simulink model "PVWDgridANN1"  (R2021a)
settings: Solver=VariableStepAuto  StartTime=0.0  StopTime=1  FixedStep=6.17283950617284E-7  MaxStep=2.0E-5  RelTol=1e-3
undefined symbols (not defined in the file): dEgdT, EgRef, gcbh, k1, Rsh_array5pc, sps_rtmsupport, Tref_K, VT_ref
libraries: neural x55, spsThreePhaseVIMeasurementLib x11, spsSeriesRLCBranchLib x9, spsVoltageMeasurementLib x7, spsDiodeLib x6, spsCurrentMeasurementLib x5, powerlib_extras x5, spsThreePhaseSeriesRLCBranchLib x4, spsThreePhaseBreakerLib x4, spsThreePhaseSeriesRLCLoadLib x3, spsUniversalBridgeLib x3, spsPVarrayModel x3
(part 1 of 7)
settings Model: Creator=Lenovo  LastModifiedBy=Sai Teja
settings SolverCC: AlgebraicLoopSolver=LineSearch
settings DebuggingCC: SFMachineParentedDataDiag=warning  ArithmeticOperatorsInVariantConditions=warning
settings ModelReferenceCC: EnableParallelModelReferenceBuilds=on  ModelReferenceMinAlgLoopOccurrences=on
settings SFSimCC: CustomCodeUndefinedFunction=UseInterfaceOnly

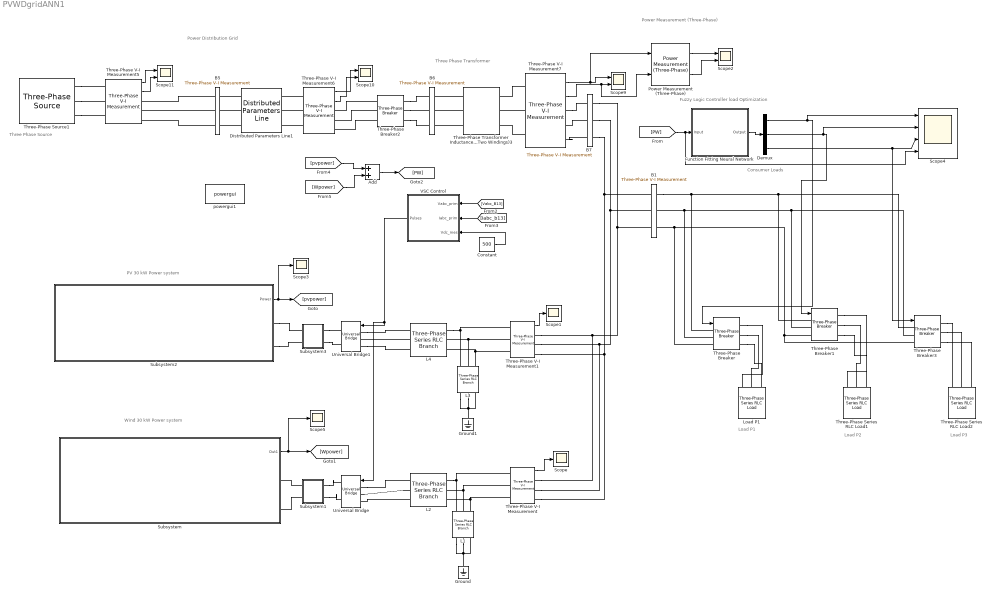
== system PVWDgridANN1 ==
  note: Fuzzy Logic Controller load Optimization
  note: Power Measurement
      | (Three-Phase)
  note: Three Phase Transformer
  note: Three Phase Source
  note: PV 30 kW Power system
  note: Load P1
  note: Power Distribution Grid
  note: Load P2
  note: Load P3
  note: Consumer Loads
  note: Wind 30 kW Power system
  Add : Sum
  B1 : spsThreePhaseVIMeasurementLib/Three-Phase V-I Measurement  VoltageMeasurement=no  SetLabelV=off  LabelV=Vabc_B13  Vpu=off  VpuLL=off  CurrentMeasurement=no  SetLabelI=off  LabelI=Iabc_b13  Ipu=off  Pbase=100e6  Vbase=440  OutputType=Magnitude  PhasorSimulation=off  PSBequivalent=0
  B5 : spsThreePhaseVIMeasurementLib/Three-Phase V-I Measurement  VoltageMeasurement=no  SetLabelV=off  LabelV=Vabc_B12  Vpu=off  VpuLL=off  CurrentMeasurement=no  SetLabelI=off  LabelI=A1  Ipu=off  Pbase=100e6  Vbase=25e3  OutputType=Magnitude  PhasorSimulation=off  PSBequivalent=0
  B6 : spsThreePhaseVIMeasurementLib/Three-Phase V-I Measurement  VoltageMeasurement=no  SetLabelV=off  LabelV=Vabc_B12  Vpu=off  VpuLL=off  CurrentMeasurement=no  SetLabelI=off  LabelI=A1  Ipu=off  Pbase=100e6  Vbase=440  OutputType=Magnitude  PhasorSimulation=off  PSBequivalent=0
  B7 : spsThreePhaseVIMeasurementLib/Three-Phase V-I Measurement  VoltageMeasurement=phase-to-ground  SetLabelV=on  LabelV=Vabc_B13  Vpu=off  VpuLL=off  CurrentMeasurement=yes  SetLabelI=on  LabelI=Iabc_b13  Ipu=off  Pbase=100e6  Vbase=440  OutputType=Magnitude  PhasorSimulation=off  PSBequivalent=0
  Constant : Constant  Value=500
  Demux : Demux  Outputs=3
  Distributed Parameters Line1 : spsDistributedParametersLineLib/Distributed Parameters Line  Phases=3  Length=100  Frequency=50  Resistance=[0.01273 0.3864]  Inductance="[0.9337e-3  4.1264e-3]"  Capacitance=[12.74e-9 7.751e-9]  x1=[-0.0006 1.14367698661715e-09 21086.3723397964 -61017.1446248442;-0.0005 1.07493118065828e-09 22992.5623173876 -60324.6973859194;-0.0004 1.00512454740211e-09 24876.0614118971 -59572.7169537636;-0.0003 9.34325977567818e-10 26735.0108371164 -58761.9454422758;-0.0002 8.62605340796205e-10 28567.5760343965 -57893.1829850521;-0.0001 7.90033416696831e-10 30371.9484831358 -56967.2869457508]  x2=[-0.0006 5.86941597339754e-09 21194.91938393 -61383.6988829109;-0.0005 5.59404825033619e-09 23112.5695475968 -60687.6612265351;-0.0004 5.31315987702939e-09 25007.4103955344 -59931.7321754389;-0.0003 5.02702805638952e-09 26877.5719485928 -59116.6577403313;-0.0002 4.73593516597845e-09 28721.2085831066 -58243.2423012745;-0.0001 4.44016847933494e-09 30536.5008523023 -57312.3478138583]  x3=[-0.0006 5.6514601122434e-11 53.1137000849838 -233.04087477199;-0.0005 5.70127645300196e-11 60.4074824530608 -231.25754153085;-0.0004 5.74546632222485e-11 67.6416499290405 -229.245985016281;-0.0003 5.78398610984626e-11 74.8090632630155 -227.008190391703;-0.0002 5.81679780148637e-11 81.9026490833576 -224.54636609024;-0.0001 5.84386901596691e-11 88.9154068772811 -221.862941635257]  x4=[-0.0006 -4.63263341454855e-11 78.0562173688537 -225.948056909574;-0.0005 -4.72451010975785e-11 85.1149013172606 -223.384760144692;-0.0004 -4.81172428388583e-11 92.089587134114 -220.601009591115;-0.0003 -4.89418986707213e-11 98.9733916465766 -217.599552474555;-0.0002 -4.97182547574234e-11 105.759521370686 -214.383350870815;-0.0001 -5.04455449292375e-11 112.441279215705 -210.955578782581]  x5=0.000565541566995743  V1=[0 0 0 1.442e-09 6.456e+04 6.456e+04;0 0 0 314.2 314.2 314.2;1.571 1.571 1.571 -0.8406 0.4129 -1.158]  V2=[0 0 0 6.152e-09 6.494e+04 6.494e+04;0 0 0 314.2 314.2 314.2;1.571 1.571 1.571 -0.9733 0.4126 -1.158]  I1=[0 0 0 3.485e-11 239 239;0 0 0 314.2 314.2 314.2;1.571 1.571 1.571 -2.244 0.3044 -1.266]  I2=[0 0 0 3.246e-11 239 239;0 0 0 314.2 314.2 314.2;1.571 1.571 1.571 0.613 0.4126 -1.158]  nHarmo=2  Measurements=None  Decoupling=off  VsMag0=0  VrMag0=0  VsAngle0=0  VrAngle0=0  IsMag0=0  IrMag0=0  IsAngle0=0  IrAngle0=0
      settings: SourceProductBaseCode=PS
  Function Fitting Neural Network : Subsystem
      mask help: Function Fitting Neural Network
      mask Display: e = 0.06;c1 = [120 150 230]/255;c2 = ([120 150 230]+0)/383;c3 = ([120 150 230]+128)/383;patch([0 1 1 0],[0 0 1 1],c1);patch([0 1 1 1-e 1-e 0+e],[0 0 1 1-e 0+e 0+e],c2);patch([0 0 1 1-e 0+e 0+e],[0 1 1 1-e 1-e 0+e],c3);plot([0 1 1 0 0],[0 0 1 1 0]);fprintf('NNET');port_label('input',1,' Input');port_label('output',1,'Output ');
  Ground : spsGroundLib/Ground  LConnTagsString=a
  Ground1 : spsGroundLib/Ground  LConnTagsString=a
  L1 : spsThreePhaseSeriesRLCBranchLib/Three-Phase Series RLC Branch  LConnTagsString=A|B|C  RConnTagsString=A|B|C  BranchType=C  Resistance=500e-6*377/50/2  Inductance=1e-2  Capacitance=100e-6  Measurements=None
  L2 : spsThreePhaseSeriesRLCBranchLib/Three-Phase Series RLC Branch  LConnTagsString=A|B|C  RConnTagsString=A|B|C  BranchType=RL  Resistance=1  Inductance=3e-2  Capacitance=900e-6  Measurements=None
  L3 : spsThreePhaseSeriesRLCBranchLib/Three-Phase Series RLC Branch  LConnTagsString=A|B|C  RConnTagsString=A|B|C  BranchType=C  Resistance=500e-6*377/50/2  Inductance=1e-2  Capacitance=100e-6  Measurements=None
  L4 : spsThreePhaseSeriesRLCBranchLib/Three-Phase Series RLC Branch  LConnTagsString=A|B|C  RConnTagsString=A|B|C  BranchType=RL  Resistance=1  Inductance=3e-2  Capacitance=900e-6  Measurements=None
  Load P1 : spsThreePhaseSeriesRLCLoadLib/Three-Phase Series RLC Load  LConnTagsString=A|B|C  Configuration=Y (grounded)  NominalVoltage=400  Vabc=[1e3 1e3 1e3]  Vabcp=[1e3 1e3 1e3]  NominalFrequency=50  UnbalancedPower=off  ActivePower=10e3  InductivePower=100  CapacitivePower=0  Pabc=[10e3 9e3 11e3]  QLabc=[100 90 110]  QCabc=[100 90 110]  Pabcp=[10e3 9e3 11e3]  QLabcp=[100 90 110]  QCabcp=[100 90 110]  Measurements=None  LoadType=constant Z
  Power Measurement (Three-Phase) : eePowerMeasurement/Power Measurement (Three-Phase)  LabelModeActiveChoice=Continuous  F=60  K=[0 1 2 3]  Seq=Positive  Ts=0
      settings: SourceProductBaseCode=PS
  Scope{,1,3,5} (4 alike) : Scope
  Scope{2,9..11} (4 alike) : Scope  NumInputPorts=2
  Scope4 : Scope  NumInputPorts=4
  Subsystem : Subsystem
  Subsystem1 : Subsystem
  Subsystem2 : Subsystem
  Subsystem3 : Subsystem
  Three-Phase Series RLC Load1 : spsThreePhaseSeriesRLCLoadLib/Three-Phase Series RLC Load  LConnTagsString=A|B|C  Configuration=Y (grounded)  NominalVoltage=400  Vabc=[1e3 1e3 1e3]  Vabcp=[1e3 1e3 1e3]  NominalFrequency=50  UnbalancedPower=off  ActivePower=10e3  InductivePower=100  CapacitivePower=0  Pabc=[10e3 9e3 11e3]  QLabc=[100 90 110]  QCabc=[100 90 110]  Pabcp=[10e3 9e3 11e3]  QLabcp=[100 90 110]  QCabcp=[100 90 110]  Measurements=None  LoadType=constant Z
  Three-Phase Series RLC Load2 : spsThreePhaseSeriesRLCLoadLib/Three-Phase Series RLC Load  LConnTagsString=A|B|C  Configuration=Y (grounded)  NominalVoltage=400  Vabc=[1e3 1e3 1e3]  Vabcp=[1e3 1e3 1e3]  NominalFrequency=50  UnbalancedPower=off  ActivePower=10e3  InductivePower=100  CapacitivePower=0  Pabc=[10e3 9e3 11e3]  QLabc=[100 90 110]  QCabc=[100 90 110]  Pabcp=[10e3 9e3 11e3]  QLabcp=[100 90 110]  QCabcp=[100 90 110]  Measurements=None  LoadType=constant Z
  Three-Phase V-I Measurement : spsThreePhaseVIMeasurementLib/Three-Phase V-I Measurement  VoltageMeasurement=phase-to-phase  SetLabelV=off  LabelV=Vabc  Vpu=off  VpuLL=off  CurrentMeasurement=no  SetLabelI=off  LabelI=Iabc  Ipu=off  Pbase=100e6  Vbase=500e3  OutputType=Complex  PhasorSimulation=off  PSBequivalent=0
  Three-Phase V-I Measurement1 : spsThreePhaseVIMeasurementLib/Three-Phase V-I Measurement  VoltageMeasurement=phase-to-phase  SetLabelV=off  LabelV=Vabc  Vpu=off  VpuLL=off  CurrentMeasurement=no  SetLabelI=off  LabelI=Iabc  Ipu=off  Pbase=100e6  Vbase=500e3  OutputType=Complex  PhasorSimulation=off  PSBequivalent=0
  Three-Phase V-I Measurement5 : spsThreePhaseVIMeasurementLib/Three-Phase V-I Measurement  VoltageMeasurement=phase-to-ground  SetLabelV=off  LabelV=Vabc  Vpu=off  VpuLL=off  CurrentMeasurement=yes  SetLabelI=off  LabelI=Iabc  Ipu=off  Pbase=100e6  Vbase=500e3  OutputType=Complex  PhasorSimulation=off  PSBequivalent=0
  Three-Phase V-I Measurement6 : spsThreePhaseVIMeasurementLib/Three-Phase V-I Measurement  VoltageMeasurement=phase-to-ground  SetLabelV=off  LabelV=Vabc  Vpu=off  VpuLL=off  CurrentMeasurement=yes  SetLabelI=off  LabelI=Iabc  Ipu=off  Pbase=100e6  Vbase=500e3  OutputType=Complex  PhasorSimulation=off  PSBequivalent=0
  Three-Phase V-I Measurement7 : spsThreePhaseVIMeasurementLib/Three-Phase V-I Measurement  VoltageMeasurement=phase-to-phase  SetLabelV=off  LabelV=Vabc_b1  Vpu=off  VpuLL=off  CurrentMeasurement=yes  SetLabelI=off  LabelI=Iabc_b1  Ipu=off  Pbase=100e6  Vbase=500e3  OutputType=Complex  PhasorSimulation=off  PSBequivalent=0
  Three-Phase Breaker : spsThreePhaseBreakerLib/Three-Phase Breaker  InitialState=open  SwitchA=on  SwitchB=on  SwitchC=on  SwitchTimes="[1/60  5/60]"  External=on  BreakerResistance=0.01  SnubberResistance=1e6  SnubberCapacitance=inf  Measurements=None
  Three-Phase Breaker1 : spsThreePhaseBreakerLib/Three-Phase Breaker  InitialState=open  SwitchA=on  SwitchB=on  SwitchC=on  SwitchTimes="[1/60  5/60]"  External=on  BreakerResistance=0.01  SnubberResistance=1e6  SnubberCapacitance=inf  Measurements=None
  Three-Phase Breaker2 : spsThreePhaseBreakerLib/Three-Phase Breaker  InitialState=closed  SwitchA=off  SwitchB=off  SwitchC=off  SwitchTimes="[1/50  20/50]"  External=off  BreakerResistance=0.001  SnubberResistance=1e6  SnubberCapacitance=inf  Measurements=None
  Three-Phase Breaker3 : spsThreePhaseBreakerLib/Three-Phase Breaker  InitialState=open  SwitchA=on  SwitchB=on  SwitchC=on  SwitchTimes="[1/60  5/60]"  External=on  BreakerResistance=0.01  SnubberResistance=1e6  SnubberCapacitance=inf  Measurements=None
  Three-Phase Source1 : spsThreePhaseSourceLib/Three-Phase Source  InternalConnection=Yg  VoltagePhases=off  Voltage=63510.4  PhaseAngle=0  Voltage_phases=[25e3 25e3 25e3]/sqrt(3)  PhaseAngles_phases=[0 -120 +120]  Frequency=50  NonIdealSource=on  SpecifyImpedance=on  Resistance=0.8929  Inductance=16.58e-3  ShortCircuitLevel=100e6  BaseVoltage=63510.4  XRratio=7  BusType=swing  Pref=0  Qref=0  Prefabc=[10e3, 10e3, 10e3]  Qrefabc=[0, 0, 0]  Qmin=-inf  Qmax=inf
  Three-Phase Transformer Inductance Matrix Type (Two Windings)3 : spsThreePhaseTransformerInductanceMatrixTypeTwoWindingsLib/Three-Phase Transformer Inductance Matrix Type (Two Windings)  CoreType=Three-limb or five-limb core  Winding1Connection=Yg  Winding2Connection=Yg  AutoTransformer=off  Measurements=None  NominalPower=[100e3 50]  VLLnom=[63510.4 254.03]  WindingResistances=[0.01 0.01]  NoLoadIexcPos=2  NoLoadPlossPos=1000  ShortCircuitReactancePos=0.06  ShortCircuitReactancePosAuto=0.06  NoLoadIexcZero=100  NoLoadPlossZero=1500  ShortCircuitReactanceZero=0.03  ShortCircuitReactanceZeroAuto=0.03
      settings: SourceProductBaseCode=PS
  Universal Bridge : spsUniversalBridgeLib/Universal Bridge  Arms=3  SnubberResistance=1e5  SnubberCapacitance=inf  Device=MOSFET / Diodes  Ron=1e-3  Lon=0  ForwardVoltages="[  0  0  ]"  ForwardVoltage=0  GTOparameters=[ 10e-6 , 20e-6 ]  IGBTparameters=[ 1e-6 , 2e-6 ]  Measurements=None  Measurements_2=None  converterType=Rectifier
  Universal Bridge1 : spsUniversalBridgeLib/Universal Bridge  Arms=3  SnubberResistance=1e5  SnubberCapacitance=inf  Device=MOSFET / Diodes  Ron=1e-3  Lon=0  ForwardVoltages="[  0  0  ]"  ForwardVoltage=0  GTOparameters=[ 10e-6 , 20e-6 ]  IGBTparameters=[ 1e-6 , 2e-6 ]  Measurements=None  Measurements_2=None  converterType=Rectifier
  VSC Control : Subsystem  mask(VSC Main Controller){nom=[ 100e3  50 ], Vnom=[ 440 440 ], Vnom_dc=440, RLxfo=[0.002  0.06 ], RLchoke=[2e-3  250e-6  ], K_VDCreg=[7  800], K_Ireg=[0.3 20], Ts=50e-6}
      mask prompts: nom "Nominal power and frequency [ Pnom(VA)  Fnom(Hz) ]:"; Vnom "Nominal primary and secondary voltages (Vrms LL) [ Vnom_prim   Vnom_sec ]:"; Vnom_dc "Nominal DC bus voltage (V):"; RLxfo "Total transformer leakage impedance (pu/Pnom) [ Rxfo  Lxf ]"; RLchoke "Choke impedance [ R(ohm) L(H) ]"; K_VDCreg "VDC regultator gains [ Kp  Ki ]:"; K_Ireg "Current regulator gains [ Kp  Ki ]:"; Ts "Sample time"
      mask init:
      | Pnom=nom(1);
      | Fnom=nom(2);
      | Vnom_prim=Vnom(1);
      | Vnom_sec=Vnom(2);
      | Zbase=Vnom_sec^2/Pnom;
      | Rtot_pu=RLxfo(1) + RLchoke(1)/Zbase;
      | Ltot_pu=RLxfo(2) + RLchoke(2)/(Zbase/(2*pi*Fnom));
      | Kp_VDCreg=K_VDCreg(1);
      | Ki_VDCreg=K_VDCreg(2);
      | Kp_Ireg=K_Ireg(1);
      | Ki_Ireg=K_Ireg(2);
      | Vdc_ref=Vnom_dc;
      | % Used to determine initial value of Boost Control (MPPT)
      | assignin('base','Vdc_ref_Inv',Vdc_ref);
  powergui1 : spspowerguiLib/powergui  Priority=1  SimulationMode=Discrete  SampleTime=1e-4  frequency=60  Iterations=50  frequencyindice=50  Pbase=100e6  ErrMax=1e-4  UnitsV=kV  UnitsW=MW  buscounter=0  FunctionMessages=off  echomessages=off  EnableUseOfTLC=off  CurrentSourceSwitches=off  DisableSnubberDevices=off  DisableRonSwitches=off  DisableVfSwitches=off  DisplayEquations=off  AutomaticDiscreteSolvers=off  SolverType=Tustin/Backward Euler (TBE)  Interpol=off  ExternalGateDelay=off  methode=off  Ts=100  x0status=blocks  SPID=on  SwTol=0  HookPort=off  NonlinearTolerance=0  nMaxIteration=15  ContinueOnMaxIteration=off  RestoreLinks=warning  ResistiveCurrentMeasurement=off  Frange=[0:2:500]  Ylog=off  Xlog=on  ShowGrid=off  save=off  variable=ZData  structure=Ctrl_Sig  ZoomFFT=off  StartTime=0.0  cycles=1  DisplayStyle=1  fundamental=60  FreqAxis=off  MaxFrequency=1000  frequencyindicesteady=1  RmsSteady=1  display=off
  wires:
  Three-Phase V-I Measurement5/2 -> Scope11/2
  Three-Phase V-I Measurement5/1 -> Scope11/1
  Three-Phase V-I Measurement7/1 -> Power Measurement (Three-Phase)/1, Scope9/1
  Three-Phase V-I Measurement6/2 -> Scope10/2
  Three-Phase V-I Measurement6/1 -> Scope10/1
  [Vabc_B13] -> VSC Control/1(Vabc_prim)
  [Iabc_b13] -> VSC Control/2(Iabc_prim)
  Constant/1 -> VSC Control/3(Vdc_mes)
  VSC Control/1(Pulses) -> Universal Bridge/1, Universal Bridge1/1
  Three-Phase V-I Measurement1/1 -> Scope1/1
  Three-Phase V-I Measurement7/2 -> Power Measurement (Three-Phase)/2, Scope9/2
  Power Measurement (Three-Phase)/1 -> Scope2/1
  Power Measurement (Three-Phase)/2 -> Scope2/2
  Function Fitting Neural Network/1(Output) -> Demux/1
  Demux/1 -> Scope4/1, Three-Phase Breaker/1
  Demux/2 -> Scope4/2, Three-Phase Breaker1/1
  Subsystem2/1(Power) -> Scope3/1, [pvpower]
  [PW] -> Scope4/4, Function Fitting Neural Network/1(Input)
  Demux/3 -> Three-Phase Breaker3/1, Scope4/3
  Subsystem/1(Out1) -> [Wpower], Scope5/1
  Three-Phase V-I Measurement/1 -> Scope/1
  [pvpower] -> Add/1
  [Wpower] -> Add/2
  Add/1 -> [PW]
  connections:
  B5/RConn2 -- Three-Phase V-I Measurement5/RConn2
  Three-Phase Breaker2/LConn2 -- B6/RConn2
  Three-Phase Source1/RConn2 -- Three-Phase V-I Measurement5/LConn2
  Three-Phase V-I Measurement7/RConn3 -- B7/RConn3
  B5/RConn1 -- Three-Phase V-I Measurement5/RConn1
  Three-Phase V-I Measurement6/LConn1 -- Distributed Parameters Line1/RConn1
  Three-Phase Breaker2/RConn3 -- Three-Phase V-I Measurement6/RConn3
  Three-Phase V-I Measurement7/LConn3 -- Three-Phase Transformer Inductance Matrix Type (Two Windings)3/RConn3
  Three-Phase V-I Measurement7/LConn2 -- Three-Phase Transformer Inductance Matrix Type (Two Windings)3/RConn2
  Three-Phase Transformer Inductance Matrix Type (Two Windings)3/LConn2 -- B6/LConn2
  Three-Phase Breaker2/LConn1 -- B6/RConn1
  Three-Phase Source1/RConn3 -- Three-Phase V-I Measurement5/LConn3
  Three-Phase V-I Measurement7/RConn2 -- B7/RConn2
  B5/RConn3 -- Three-Phase V-I Measurement5/RConn3
  Three-Phase V-I Measurement6/LConn3 -- Distributed Parameters Line1/RConn3
  Distributed Parameters Line1/LConn2 -- B5/LConn2
  Three-Phase Breaker2/RConn2 -- Three-Phase V-I Measurement6/RConn2
  Distributed Parameters Line1/LConn3 -- B5/LConn3
  Three-Phase V-I Measurement6/LConn2 -- Distributed Parameters Line1/RConn2
  Distributed Parameters Line1/LConn1 -- B5/LConn1
  Three-Phase Source1/RConn1 -- Three-Phase V-I Measurement5/LConn1
  Three-Phase V-I Measurement7/RConn1 -- B7/RConn1
  Three-Phase Breaker2/RConn1 -- Three-Phase V-I Measurement6/RConn1
  Three-Phase Transformer Inductance Matrix Type (Two Windings)3/LConn1 -- B6/LConn1
  Three-Phase Breaker2/LConn3 -- B6/RConn3
  Three-Phase Transformer Inductance Matrix Type (Two Windings)3/LConn3 -- B6/LConn3
  Three-Phase V-I Measurement7/LConn1 -- Three-Phase Transformer Inductance Matrix Type (Two Windings)3/RConn1
  B7/LConn3 -- Three-Phase V-I Measurement/RConn3 -- Three-Phase V-I Measurement1/RConn3 -- B1/RConn1
  B7/LConn2 -- Three-Phase V-I Measurement/RConn2 -- Three-Phase V-I Measurement1/RConn2 -- B1/RConn2
  B7/LConn1 -- Three-Phase V-I Measurement/RConn1 -- Three-Phase V-I Measurement1/RConn1 -- B1/RConn3
  L3/LConn3 -- Three-Phase V-I Measurement1/LConn3 -- L4/RConn3
  L3/LConn1 -- L4/RConn1 -- Three-Phase V-I Measurement1/LConn1
  L3/LConn2 -- Three-Phase V-I Measurement1/LConn2 -- L4/RConn2
  L3/RConn1 -- Ground1/LConn1 -- L3/RConn3 -- L3/RConn2
  L4/LConn2 -- Universal Bridge1/LConn2
  Universal Bridge1/LConn3 -- L4/LConn3
  Subsystem3/RConn1 -- Universal Bridge1/RConn1
  Subsystem3/RConn2 -- Universal Bridge1/RConn2
  Universal Bridge1/LConn1 -- L4/LConn1
  Subsystem2/RConn1 -- Subsystem3/LConn1
  Subsystem2/RConn2 -- Subsystem3/LConn2
  Three-Phase Breaker/RConn1 -- Load P1/LConn1
  Three-Phase Breaker/RConn2 -- Load P1/LConn2
  Three-Phase Breaker/RConn3 -- Load P1/LConn3
  Three-Phase Breaker1/RConn3 -- Three-Phase Series RLC Load1/LConn3
  Three-Phase Breaker1/RConn1 -- Three-Phase Series RLC Load1/LConn1
  Three-Phase Breaker1/RConn2 -- Three-Phase Series RLC Load1/LConn2
  Three-Phase Breaker3/RConn1 -- Three-Phase Series RLC Load2/LConn1
  Three-Phase Breaker3/RConn3 -- Three-Phase Series RLC Load2/LConn3
  Three-Phase Breaker3/RConn2 -- Three-Phase Series RLC Load2/LConn2
  B1/LConn1 -- Three-Phase Breaker/LConn1 -- Three-Phase Breaker1/LConn1 -- Three-Phase Breaker3/LConn1
  Three-Phase Breaker3/LConn2 -- Three-Phase Breaker1/LConn2 -- Three-Phase Breaker/LConn2 -- B1/LConn2
  Three-Phase Breaker3/LConn3 -- Three-Phase Breaker/LConn3 -- B1/LConn3 -- Three-Phase Breaker1/LConn3
  L2/RConn2 -- L1/LConn2 -- Three-Phase V-I Measurement/LConn2
  L2/RConn3 -- L1/LConn3 -- Three-Phase V-I Measurement/LConn3
  L1/LConn1 -- L2/RConn1 -- Three-Phase V-I Measurement/LConn1
  L1/RConn3 -- L1/RConn1 -- Ground/LConn1 -- L1/RConn2
  Subsystem1/LConn2 -- Subsystem/RConn2
  Subsystem1/RConn1 -- Universal Bridge/RConn1
  Subsystem1/LConn1 -- Subsystem/RConn1
  Universal Bridge/LConn1 -- L2/LConn1
  Subsystem1/RConn2 -- Universal Bridge/RConn2
  L2/LConn2 -- Universal Bridge/LConn2
  Universal Bridge/LConn3 -- L2/LConn3

== system PVWDgridANN1/Function Fitting Neural Network ==
  Input : Inport  PortDimensions=1
      mask Display: e = 0.06;c1 = [120 230 180]/255;c2 = ([120 230 180]+0)/(256+128);c3 = ([120 230 180]+128)/(256+128);patch([0 1 1 0],[0 0 1 1],c1);patch([0 1 1 1-e 1-e 0+e],[0 0 1 1-e 0+e 0+e],c2);patch([0 0 1 1-e 0+e 0+e],[0 1 1 1-e 1-e 0+e],c3);plot([0 1 1 0 0],[0 0 1 1 0]);
  Layer 1 : Subsystem
      mask Display: e = 0.06;c1 = [120 150 230]/255;c2 = ([120 150 230]+0)/383;c3 = ([120 150 230]+128)/383;patch([0 1 1 0],[0 0 1 1],c1);patch([0 1 1 1-e 1-e 0+e],[0 0 1 1-e 0+e 0+e],c2);patch([0 0 1 1-e 0+e 0+e],[0 1 1 1-e 1-e 0+e],c3);plot([0 1 1 0 0],[0 0 1 1 0]);
  Layer 2 : Subsystem
      mask Display: e = 0.06;c1 = [120 150 230]/255;c2 = ([120 150 230]+0)/383;c3 = ([120 150 230]+128)/383;patch([0 1 1 0],[0 0 1 1],c1);patch([0 1 1 1-e 1-e 0+e],[0 0 1 1-e 0+e 0+e],c2);patch([0 0 1 1-e 0+e 0+e],[0 1 1 1-e 1-e 0+e],c3);plot([0 1 1 0 0],[0 0 1 1 0]);
  Process Input 1 : Subsystem
      mask Display: e = 0.06;c1 = [120 150 230]/255;c2 = ([120 150 230]+0)/383;c3 = ([120 150 230]+128)/383;patch([0 1 1 0],[0 0 1 1],c1);patch([0 1 1 1-e 1-e 0+e],[0 0 1 1-e 0+e 0+e],c2);patch([0 0 1 1-e 0+e 0+e],[0 1 1 1-e 1-e 0+e],c3);plot([0 1 1 0 0],[0 0 1 1 0]);
  Output : Outport  InitialOutput=[0;0;0]
      mask Display: e = 0.06;c1 = [120 230 180]/255;c2 = ([120 230 180]+0)/(256+128);c3 = ([120 230 180]+128)/(256+128);patch([0 1 1 0],[0 0 1 1],c1);patch([0 1 1 1-e 1-e 0+e],[0 0 1 1-e 0+e 0+e],c2);patch([0 0 1 1-e 0+e 0+e],[0 1 1 1-e 1-e 0+e],c3);plot([0 1 1 0 0],[0 0 1 1 0]);
  wires:
  Input/1 -> Process Input 1/1(x)
  Layer 2/1("a{2}") -> Output/1
  Process Input 1/1(p) -> Layer 1/1("p{1}")
  Layer 1/1("a{1}") -> [feedback1]
  [feedback1] -> Layer 2/1("a{1} ")

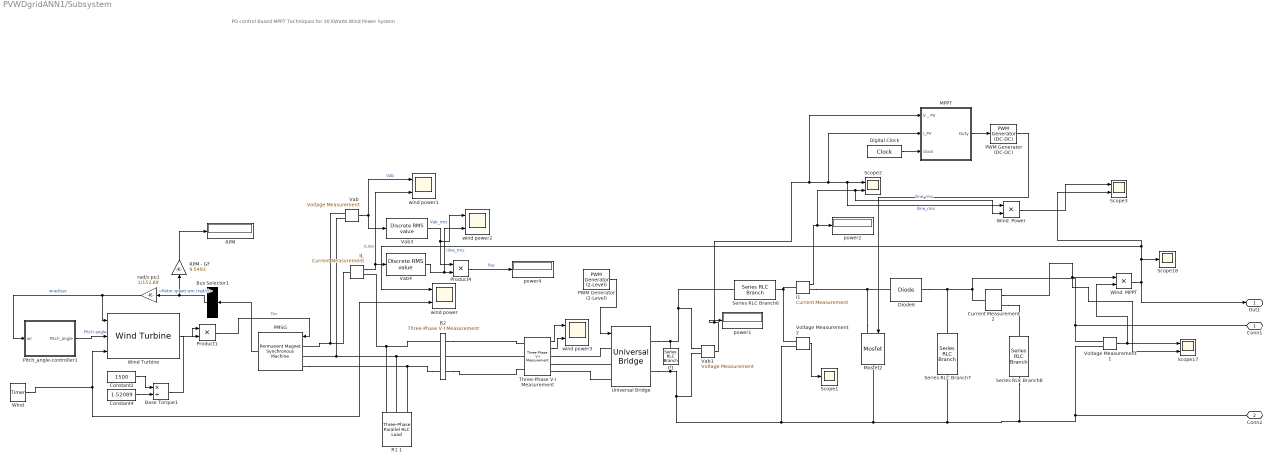
== system PVWDgridANN1/Subsystem ==
  note: PO control Based MPPT Techniques for 30 KWatts Wind Power System
  "B2 " : spsThreePhaseVIMeasurementLib/Three-Phase V-I Measurement  VoltageMeasurement=no  SetLabelV=on  LabelV=Vabc_B2  Vpu=off  VpuLL=off  CurrentMeasurement=no  SetLabelI=on  LabelI=Iabc_B2  Ipu=off  Pbase=100e6  Vbase=500e3  OutputType=Magnitude  PhasorSimulation=off  PSBequivalent=0
  Base Torque1 : Product  Inputs=*/  RndMeth=Zero
  Bus Selector1 : BusSelector  OutputSignals=Rotor speed wm (rad/s)
  C1 : spsSeriesRLCBranchLib/Series RLC Branch  LConnTagsString=__new0  RConnTagsString=__new0  BranchType=C  Resistance=0.001  Inductance=1e-3  SetiL0=off  InitialCurrent=0  Capacitance=900e-6  Setx0=off  InitialVoltage=0  Measurements=None
  Constant2 : Constant  Value=1500
  Constant4 : Constant  Value=1.52089
  Current Measurement2 : spsCurrentMeasurementLib/Current Measurement  PhasorSimulation=off  OutputType=Complex  PSBequivalent=0
  Digital Clock : DigitalClock  SampleTime=0.001
  Diode6 : spsDiodeLib/Diode  Ron=0.001  Lon=0  Vf=0.8  IC=0  UseSnubber=0  Rs=500  Cs=250e-9  Measurements=off
  I1 : spsCurrentMeasurementLib/Current Measurement  PhasorSimulation=off  OutputType=Complex  PSBequivalent=0
  IL : spsCurrentMeasurementLib/Current Measurement  PhasorSimulation=off  OutputType=Complex  PSBequivalent=0
  MPPT : Subsystem
  Mosfet2 : spsMosfetLib/Mosfet  Ron=0.1  Lon=0  Rd=0.01  Vfd=0.8  IC=0  Rs=1e5  Cs=inf  Measurements=off
  PMSG : spsPermanentMagnetSynchronousMachineLib/Permanent Magnet Synchronous Machine  NbPhases=3  FluxDistribution=Sinusoidal  RotorType=Round  MechanicalLoad=Torque Tm  PresetModel="16:  111 Nm 560 Vdc 3000 RPM - 126 Nm"  ShowDetailedParameters=on  MeasurementBus=off  Resistance=0.05  Inductance=8.5e-3  dqInductances=[0.0082 0.0082]  La=0.000635  MachineConstant=Flux linkage established by magnets (V.s)  Flux=0.192  VoltageCst=139.2998  TorqueCst=1.152  Flat=120  Mechanical=[0.011 0.001889 4 0]  PolePairs=4  InitialConditions=[0,0, 0,0]  InitialConditions5ph=[0 0 0 0 0 0]  RefAngle=90 degrees behind phase A axis (modified Park)  IterativeDiscreteModel=Trapezoidal non iterative  TsBlock=-1  TsPowergui=0
  PWM Generator (2-Level) : spsPWMGenerator2LevelLib/PWM Generator (2-Level)  ModulatorType=Three-phase bridge (6 pulses)  ModulatorMode=Unsynchronized  Fc=3000  Pc=90  nF=27  MinMax="[ -1  1 ]"  SamplingTechnique=Natural  ModulatingSignals=on  m=0.8  Freq=50  Phase=0  Ts=0  ShowCarrierOutport=off
  PWM Generator (DC-DC) : spsPWMGeneratorDCDCLib/PWM Generator (DC-DC)  Fsw=5000  Ts=0
  Pitch_angle-controller1 : Subsystem
  Product1 : Product  RndMeth=Zero
  Product4 : Product  RndMeth=Zero
  R1 1 : spsThreePhaseParallelRLCLoadLib/Three-Phase Parallel RLC Load  LConnTagsString=A|B|C  Configuration=Y (grounded)  NominalVoltage=220  Vabc=[1e3 1e3 1e3]  Vabcp=[1e3 1e3 1e3]  NominalFrequency=50  UnbalancedPower=off  ActivePower=5000  InductivePower=0  CapacitivePower=0  Pabc=[9e3 9e3 9e3]  QLabc=[100 90 110]  QCabc=[100 90 110]  Pabcp=[10e3 9e3 11e3]  QLabcp=[100 90 110]  QCabcp=[100 90 110]  Measurements=None  LoadType=constant Z
  "RPM " : Display
  RPM - GF : Gain  Gain=9.5493  SaturateOnIntegerOverflow=on  OutDataTypeStr=Inherit: Same as input  ParamDataTypeStr=Inherit: Same as input
  Scope1 : Scope
  Scope17 : Scope  NumInputPorts=2
  Scope18 : Scope
  Scope2 : Scope  NumInputPorts=2
  Scope3 : Scope  NumInputPorts=2
  Series RLC Branch6 : spsSeriesRLCBranchLib/Series RLC Branch  LConnTagsString=__new0  RConnTagsString=__new0  BranchType=L  Resistance=1  Inductance=0.4e-1  SetiL0=off  InitialCurrent=0  Capacitance=1e-6  Setx0=off  InitialVoltage=0  Measurements=None
  Series RLC Branch7 : spsSeriesRLCBranchLib/Series RLC Branch  LConnTagsString=__new0  RConnTagsString=__new0  BranchType=C  Resistance=110  Inductance=1e-3  SetiL0=off  InitialCurrent=0  Capacitance=750e-6  Setx0=off  InitialVoltage=0  Measurements=None
  Series RLC Branch8 : spsSeriesRLCBranchLib/Series RLC Branch  LConnTagsString=__new0  RConnTagsString=__new0  BranchType=R  Resistance=6  Inductance=1e-3  SetiL0=off  InitialCurrent=0  Capacitance=1e-6  Setx0=off  InitialVoltage=0  Measurements=None
  Three-Phase V-I Measurement : spsThreePhaseVIMeasurementLib/Three-Phase V-I Measurement  VoltageMeasurement=phase-to-phase  SetLabelV=off  LabelV=Vabc  Vpu=off  VpuLL=off  CurrentMeasurement=yes  SetLabelI=off  LabelI=Iabc  Ipu=off  Pbase=100e6  Vbase=500e3  OutputType=Complex  PhasorSimulation=off  PSBequivalent=0
  Universal Bridge : spsUniversalBridgeLib/Universal Bridge  Arms=3  SnubberResistance=1e5  SnubberCapacitance=inf  Device=Thyristors  Ron=1e-3  Lon=0  ForwardVoltages="[  0  0  ]"  ForwardVoltage=0.8  GTOparameters=[ 10e-6 , 20e-6 ]  IGBTparameters=[ 1e-6 , 2e-6 ]  Measurements=None  Measurements_2=None  converterType=Rectifier
  Vab : spsVoltageMeasurementLib/Voltage Measurement  PhasorSimulation=off  OutputType=Complex  PSBequivalent=0
  Vab1 : spsVoltageMeasurementLib/Voltage Measurement  PhasorSimulation=off  OutputType=Complex  PSBequivalent=0
  Vab3 : powerlib_extras/Discrete Measurements/Discrete  RMS value  Freq=50  Mag_Init=0  Ts=20e-6
      settings: SourceProductBaseCode=PS
  Vab4 : powerlib_extras/Discrete Measurements/Discrete  RMS value  Freq=50  Mag_Init=0  Ts=20e-6
      settings: SourceProductBaseCode=PS
  Voltage Measurement1 : spsVoltageMeasurementLib/Voltage Measurement  PhasorSimulation=off  OutputType=Complex  PSBequivalent=0
  Voltage Measurement2 : spsVoltageMeasurementLib/Voltage Measurement  PhasorSimulation=off  OutputType=Complex  PSBequivalent=0
  "Wind " : powerlib_extras/Control  Blocks/Timer  t=[0 0.05 0.1 0.15 0.2 ]  e=[5 7 11 12 12]
      settings: SourceProductBaseCode=PS
  "Wind  MPPT " : Product
  Wind  Power : Product
  Wind Turbine : spsWindTurbineLib/Wind Turbine  Pnom=80000  Pelec_base=80000/0.9  wind_base=12  P_wind_base=0.73  speed_nom=1.2  pitch_angle=0  c1_c6="[0.51763          116          0.4            5           21     0.006795]"  cp_nom=0.48  lambda_nom=8.1
      settings: SourceProductBaseCode=PS
  power1 : Display
      settings: SampleTime=1e-3
  power2 : Display
      settings: SampleTime=1e-3
  power4 : Display
      settings: SampleTime=1e-3
  rad/s pu1 : Gain  Gain=1/152.89  SaturateOnIntegerOverflow=on  OutDataTypeStr=Inherit: Same as input  ParamDataTypeStr=Inherit: Same as input
  wind power{,1..3} (4 alike) : Scope  NumInputPorts=2
  Conn1 : PMIOPort  Side=Right
  Conn2 : PMIOPort  Port=2  Side=Right
  Out1 : Outport  VectorParamsAs1DForOutWhenUnconnected=off
  wires:
  Product4/1 -> power4/1  "Pac"
  "Wind  MPPT "/1 -> wind power/1, Scope3/2, Scope18/1, Out1/1
  Current Measurement2/1 -> Scope17/2, "Wind  MPPT "/1
  Vab3/1 -> Product4/1, wind power2/1  "Vab_rms"
  IL/1 -> Vab4/1, wind power1/2  "ILine"
  Digital Clock/1 -> MPPT/3(clock)
  MPPT/1(Duty) -> PWM Generator (DC-DC)/1
  Wind  Power/1 -> Scope3/1
  Base Torque1/1 -> Product1/2
  Vab/1 -> Vab3/1, wind power1/1  "Vab"
  Wind Turbine/1 -> Product1/1
  PWM Generator (2-Level)/1 -> Universal Bridge/1
  Pitch_angle-controller1/1(Pitch_angle) -> Wind Turbine/2  "Pitch angle"
  "Wind "/1 -> Wind Turbine/3, wind power/2
  Constant2/1 -> Base Torque1/1
  PWM Generator (DC-DC)/1 -> Mosfet2/1
  Bus Selector1/1 -> RPM - GF/1, rad/s pu1/1  "<Rotor speed wm (rad/s)>"
  PMSG/1 -> Bus Selector1/1
  I1/1 -> Wind  Power/2, Scope2/2, power2/1  "Iline_rms"
  rad/s pu1/1 -> Wind Turbine/1, Pitch_angle-controller1/1(wr)  "wrad/sec"
  Constant4/1 -> Base Torque1/2
  Three-Phase V-I Measurement/1 -> wind power3/1
  Vab1/1 -> power1/1, MPPT/1("V _ PV "), MPPT/2(I_PV), Wind  Power/1, Scope2/1  "Iline_rms"
  Product1/1 -> PMSG/1  "Tm"
  Vab4/1 -> wind power2/2, Product4/2  "Iline_rms"
  Voltage Measurement2/1 -> Scope1/1
  Voltage Measurement1/1 -> "Wind  MPPT "/2, Scope17/1
  Three-Phase V-I Measurement/2 -> wind power3/2
  RPM - GF/1 -> "RPM "/1
  connections:
  IL/RConn1 -- "B2 "/LConn1 -- R1 1/LConn1
  Three-Phase V-I Measurement/RConn2 -- Universal Bridge/LConn2
  PMSG/LConn2 -- Vab/LConn2 -- "B2 "/LConn2 -- R1 1/LConn2
  IL/LConn1 -- Vab/LConn1 -- PMSG/LConn1
  Voltage Measurement1/LConn1 -- Series RLC Branch7/LConn1 -- Diode6/RConn1 -- Current Measurement2/LConn1 -- Conn1/RConn1
  Series RLC Branch8/RConn1 -- Conn2/RConn1 -- Voltage Measurement1/LConn2 -- C1/RConn1 -- Universal Bridge/RConn2 -- Vab1/LConn2 -- Voltage Measurement2/LConn2 -- Mosfet2/RConn1 -- Series RLC Branch7/RConn1
  Voltage Measurement2/LConn1 -- Series RLC Branch6/RConn1 -- I1/LConn1
  Vab1/LConn1 -- Series RLC Branch6/LConn1 -- C1/LConn1 -- Universal Bridge/RConn1
  Three-Phase V-I Measurement/RConn3 -- Universal Bridge/LConn3
  "B2 "/LConn3 -- PMSG/LConn3 -- R1 1/LConn3
  Mosfet2/LConn1 -- I1/RConn1 -- Diode6/LConn1
  Three-Phase V-I Measurement/RConn1 -- Universal Bridge/LConn1
  "B2 "/RConn3 -- Three-Phase V-I Measurement/LConn3
  Three-Phase V-I Measurement/LConn2 -- "B2 "/RConn2
  "B2 "/RConn1 -- Three-Phase V-I Measurement/LConn1
  Current Measurement2/RConn1 -- Series RLC Branch8/LConn1

== system PVWDgridANN1/Subsystem1 ==
  Diode : spsDiodeLib/Diode  Ron=0.001  Lon=0  Vf=0.8  IC=0  UseSnubber=0  Rs=500  Cs=250e-9  Measurements=off
  Diode1 : spsDiodeLib/Diode  Ron=0.001  Lon=0  Vf=0.8  IC=0  UseSnubber=0  Rs=500  Cs=250e-9  Measurements=off
  1 : PMIOPort  Side=Left
  2 : PMIOPort  Port=2  Side=Right
  3 : PMIOPort  Port=3  Side=Left
  4 : PMIOPort  Port=4  Side=Right
  connections:
  Diode1/LConn1 -- 3/RConn1
  Diode/LConn1 -- 1/RConn1
  Diode1/RConn1 -- 4/RConn1
  Diode/RConn1 -- 2/RConn1
